simulink model "sm_tVtest_belt_trackSeg"  (R2026a)
settings: Solver=ode23t  StopTime=2.5  AbsTol=1e-3  EnableMultiTasking=on
undefined symbols (not defined in the file or in its folder): Trac, track_seg_tgts_seg25i2u0r3, X, Y, Z
libraries: sm_lib x9, sm_trackV_lib_belt_contact_internal_sets x3, sm_trackV_lib_belt_contact x3, sm_trackV_lib_belt_underc_elem x3, sm_trackV_lib_belt_segment x3, nesl_utility x1
Description:
  | Belt Track Segments
  | Copyright 2024-2026 The MathWorks, Inc.
settings Model: Creator=smiller  LastModifiedBy=smiller
settings DebuggingCC: SubsystemReferenceDiagnosticForUnitTest=warning
settings SimscapeCC: SimscapeNominalValues="[{\"value\":\"1\",\"unit\":\"A\"},{\"value\":\"1\",\"unit\":\"bar\"},{\"value\":\"1\",\"unit\":\"cm^2\"},{\"value\":\"1\",\"unit\":\"cm^3/s\"},{\"value\":\"1\",\"unit\":\"kJ/kg\"},{\"value\":\"1\",\"unit\":\"kW\"},{\"value\":\"1\",\"unit\":\"l\"},{\"value\":\"1\",\"unit\":\"N\"},{\"value\":\"1\",\"unit\":\"N*m\"},{\"value\":\"1\",\"unit\":\"V\"}]"  SimscapeLogSimulationStatistics=on
settings ExplorerConfigSet: InternalSimMechanicsExplorerSettings="<ExplorerConfiguration><canonicalview>default</canonicalview><AnimationSetting><BasePlaybackSpeed>1.0</BasePlaybackSpeed><PlaybackSpeedFactor>1.0</PlaybackSpeedFactor></AnimationSetting><TilePanel><TileInfo><Tiles Columns=\"1\" Count=\"1\" Rows=\"1\"><Column Weight=\"1\"/><Row Weight=\"1\"/><Tile Height=\"1\" Width=\"1\" X=\"0\" Y=\"0\"/></Tiles></TileInfo><SceneInfo><SceneViewer><BGColor><R>1</R><G>1</G><B>1</B></BGColor><Camera><DoPerspective>off</DoPerspective><Position><X>0.0792342818112368175</X><Y>-1.47217004076199931</Y><Z>-0.215028231058741581</Z></Position><Center><X>-0.384436321912249857</X><Y>-0.0022500717732171216</Y><Z>-0.342061483853710324</Z></Center><Up><X>0.00408619380834399082</X><Y>0.0873795501498821903</Y><Z>0.996166711567780361</Z></Up><ViewLimDist>1</ViewLimDist><YLim>0.935866935253143351</YLim><XLim>1.10917562696668837</XLim></Camera></SceneViewer></SceneInfo></TilePanel><MechEditorPanel><Cameras/><GfxPanelCameraMap/><VideoCreator><PlaybackSpeedRatio>1.0</PlaybackSpeedRatio><FrameRate>30</FrameRate><VideoFormat>Motion JPEG AVI</VideoFormat><FrameSize>auto</FrameSize></VideoCreator></MechEditorPanel></ExplorerConfiguration>"

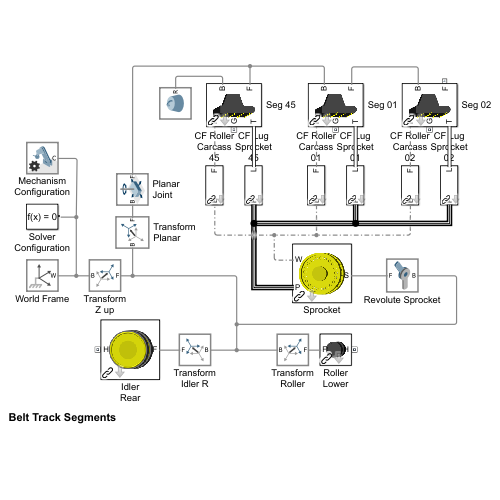
[thumbnail: Simulink's stored preview of the top-level diagram]
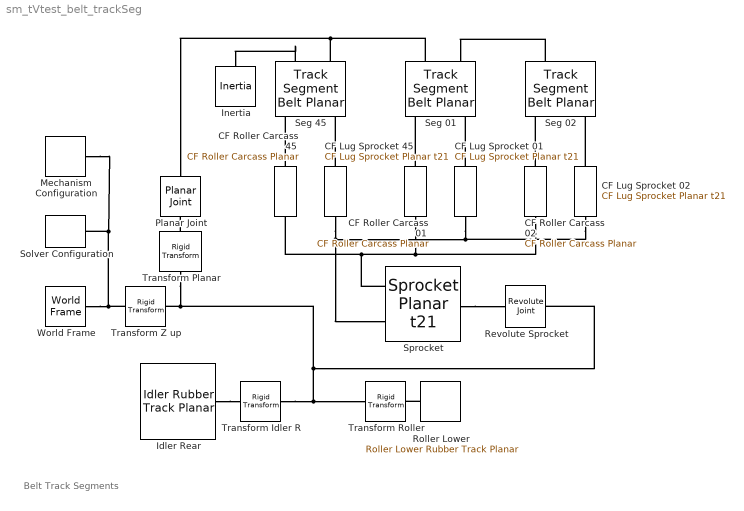
== system sm_tVtest_belt_trackSeg ==
  note: Belt Track Segments
  CF Lug Sprocket 01 : sm_trackV_lib_belt_contact_internal_sets/CF Lug Sprocket Planar t21  K_SprocketLug=Trac.Contact.SprocketLug.K  B_SprocketLug=Trac.Contact.SprocketLug.B  TW_SprocketLug=Trac.Contact.SprocketLug.TW
  CF Lug Sprocket 02 : sm_trackV_lib_belt_contact_internal_sets/CF Lug Sprocket Planar t21  K_SprocketLug=Trac.Contact.SprocketLug.K  B_SprocketLug=Trac.Contact.SprocketLug.B  TW_SprocketLug=Trac.Contact.SprocketLug.TW
  CF Lug Sprocket 45 : sm_trackV_lib_belt_contact_internal_sets/CF Lug Sprocket Planar t21  K_SprocketLug=Trac.Contact.SprocketLug.K  B_SprocketLug=Trac.Contact.SprocketLug.B  TW_SprocketLug=Trac.Contact.SprocketLug.TW
  CF Roller Carcass 01 : sm_trackV_lib_belt_contact/CF Roller Carcass Planar  K_Roller=Trac.Contact.SprocketRoller.K  B_Roller=Trac.Contact.SprocketRoller.B  TW_Roller=Trac.Contact.SprocketRoller.TW
  CF Roller Carcass 02 : sm_trackV_lib_belt_contact/CF Roller Carcass Planar  K_Roller=Trac.Contact.SprocketRoller.K  B_Roller=Trac.Contact.SprocketRoller.B  TW_Roller=Trac.Contact.SprocketRoller.TW
  CF Roller Carcass 45 : sm_trackV_lib_belt_contact/CF Roller Carcass Planar  K_Roller=Trac.Contact.SprocketRoller.K  B_Roller=Trac.Contact.SprocketRoller.B  TW_Roller=Trac.Contact.SprocketRoller.TW
  Idler Rear : sm_trackV_lib_belt_underc_elem/Idler Rubber Track Planar  idler_rad=Trac.IdlerR.rad  idler_len=Trac.IdlerR.len  wheel_clr=Trac.IdlerR.Wheel.clr  rim_rad=Trac.IdlerR.Rim.rad  rim_hub_rad=Trac.IdlerF.Rim.hub_rad  rim_xc=Trac.IdlerR.Rim.rim_xc  idler_rho=Trac.IdlerR.rho  idler_opc=Trac.IdlerR.opc  idler_clr=Trac.IdlerR.clr  idler_axle_rad=Trac.IdlerR.Axle.rad  idler_axle_len=Trac.IdlerR.Axle.len  idler_axle_rho=Trac.IdlerR.Axle.rho  idler_axle_opc=Trac.IdlerR.Axle.opc  idler_axle_clr=Trac.IdlerR.Axle.clr  idler_contgeo_clr=Trac.IdlerR.belt_contact.clr  idler_contgeo_opc=Trac.IdlerR.belt_contact.opc
  Inertia : sm_lib/Body Elements/Inertia  InertiaType=Custom  Mass=Trac.Belt.mass  MassUnits=kg  CenterOfMass=[0 0 0]  CenterOfMassUnits=m  MomentsOfInertia=[1 1 1]  MomentsOfInertiaUnits=kg*m^2  ProductsOfInertia=[0 0 0]  ProductsOfInertiaUnits=kg*m^2  GraphicType=None  MarkerShape=Inertia  MarkerSize=20  GraphicVisPropType=SimpleVisualProperties  GraphicDiffuseColor=[0.5 0.5 0.5]  GraphicOpacity=1.0  GraphicSpecularColor=[0.5 0.5 0.5 1.0]  GraphicAmbientColor=[0.15 0.15 0.15 1.0]  GraphicEmissiveColor=[0.0 0.0 0.0 1.0]  GraphicShininess=75
  Mechanism Configuration : sm_lib/Utilities/Mechanism Configuration  UniformGravity=Constant  GravityVector=[0 0 -9.80665]  GravityVectorUnits=m/s^2  LinearizationDelta=0.001  JointModeTransitionNonlinearIterations=2
  Planar Joint : sm_lib/Joints/Planar Joint  JointMode=Normal  CompositeWrenchDir=FollowerOnBase  CompositeWrenchFrame=BaseFrame  SenseConstraintForce=off  SenseConstraintTorque=off  SenseTotalForce=off  SenseTotalTorque=off  PxPositionTargetSpecify=off  PxPositionTargetPriority=High  PxPositionTargetValue=0  PxPositionTargetValueUnits=m  PxVelocityTargetSpecify=off  PxVelocityTargetPriority=High  PxVelocityTargetValue=0  PxVelocityTargetValueUnits=m/s  PxEquilibriumPosition=0  PxEquilibriumPositionUnits=m  PxSpringStiffness=0  PxSpringStiffnessUnits=N/m  PxDampingCoefficient=0  PxDampingCoefficientUnits=N/(m/s)  PxLowerLimitSpecify=off  PxLowerLimitBound=-1  PxLowerLimitBoundUnits=m  PxLowerLimitStiffness=1e6  PxLowerLimitStiffnessUnits=N/m  PxLowerLimitDamping=1e3  PxLowerLimitDampingUnits=N/(m/s)  PxLowerLimitTransitionRegionWidth=1e-4  PxLowerLimitTransitionRegionWidthUnits=m  PxUpperLimitSpecify=off  PxUpperLimitBound=1  PxUpperLimitBoundUnits=m  PxUpperLimitStiffness=1e6  PxUpperLimitStiffnessUnits=N/m  PxUpperLimitDamping=1e3  PxUpperLimitDampingUnits=N/(m/s)  PxUpperLimitTransitionRegionWidth=1e-4  PxUpperLimitTransitionRegionWidthUnits=m  PxTorqueActuationMode=NoTorque  PxMotionActuationMode=ComputedMotion  PxSensePosition=off  PxSenseVelocity=off  PxSenseAcceleration=off  PxSenseTorqueForce=off  PxSenseLowerLimitTorqueForce=off  PxSenseUpperLimitTorqueForce=off  PyPositionTargetSpecify=off  PyPositionTargetPriority=High  PyPositionTargetValue=0  PyPositionTargetValueUnits=m  PyVelocityTargetSpecify=off  PyVelocityTargetPriority=High  PyVelocityTargetValue=0  PyVelocityTargetValueUnits=m/s  PyEquilibriumPosition=0  PyEquilibriumPositionUnits=m  PySpringStiffness=0  PySpringStiffnessUnits=N/m  PyDampingCoefficient=0  PyDampingCoefficientUnits=N/(m/s)  PyLowerLimitSpecify=off  PyLowerLimitBound=-1  PyLowerLimitBoundUnits=m  PyLowerLimitStiffness=1e6  PyLowerLimitStiffnessUnits=N/m  PyLowerLimitDamping=1e3  PyLowerLimitDampingUnits=N/(m/s)  PyLowerLimitTransitionRegionWidth=1e-4  PyLowerLimitTransitionRegionWidthUnits=m  PyUpperLimitSpecify=off  PyUpperLimitBound=1  PyUpperLimitBoundUnits=m  PyUpperLimitStiffness=1e6  PyUpperLimitStiffnessUnits=N/m  PyUpperLimitDamping=1e3  PyUpperLimitDampingUnits=N/(m/s)  PyUpperLimitTransitionRegionWidth=1e-4  PyUpperLimitTransitionRegionWidthUnits=m  PyTorqueActuationMode=NoTorque  PyMotionActuationMode=ComputedMotion  PySensePosition=off  PySenseVelocity=off  PySenseAcceleration=off  PySenseTorqueForce=off  PySenseLowerLimitTorqueForce=off  PySenseUpperLimitTorqueForce=off  RzPositionTargetSpecify=on  RzPositionTargetPriority=High  RzPositionTargetValue=0  RzPositionTargetValueUnits=deg  RzVelocityTargetSpecify=off  RzVelocityTargetPriority=High  RzVelocityTargetValue=0  RzVelocityTargetValueUnits=deg/s  RzEquilibriumPosition=0  RzEquilibriumPositionUnits=deg  RzSpringStiffness=0  RzSpringStiffnessUnits=N*m/deg  RzDampingCoefficient=0  RzDampingCoefficientUnits=N*m/(deg/s)  RzLowerLimitSpecify=off  RzLowerLimitBound=-90  RzLowerLimitBoundUnits=deg  RzLowerLimitStiffness=1e4  RzLowerLimitStiffnessUnits=N*m/deg  RzLowerLimitDamping=10  RzLowerLimitDampingUnits=N*m/(deg/s)  RzLowerLimitTransitionRegionWidth=0.1  RzLowerLimitTransitionRegionWidthUnits=deg  RzUpperLimitSpecify=off  RzUpperLimitBound=90  RzUpperLimitBoundUnits=deg  RzUpperLimitStiffness=1e4  RzUpperLimitStiffnessUnits=N*m/deg  RzUpperLimitDamping=10  RzUpperLimitDampingUnits=N*m/(deg/s)  RzUpperLimitTransitionRegionWidth=0.1  RzUpperLimitTransitionRegionWidthUnits=deg  RzTorqueActuationMode=NoTorque  RzMotionActuationMode=ComputedMotion  RzSensePosition=off  RzSenseVelocity=off  RzSenseAcceleration=off  RzSenseTorqueForce=off  RzSenseLowerLimitTorqueForce=off  RzSenseUpperLimitTorqueForce=off
  Revolute Sprocket : sm_lib/Joints/Revolute Joint  JointMode=Normal  CompositeWrenchDir=FollowerOnBase  CompositeWrenchFrame=BaseFrame  SenseConstraintForce=off  SenseConstraintTorque=off  SenseTotalForce=off  SenseTotalTorque=off  PositionTargetSpecify=off  PositionTargetPriority=High  PositionTargetValue=0  PositionTargetValueUnits=deg  VelocityTargetSpecify=off  VelocityTargetPriority=High  VelocityTargetValue=0  VelocityTargetValueUnits=deg/s  EquilibriumPosition=0  EquilibriumPositionUnits=deg  SpringStiffness=0  SpringStiffnessUnits=N*m/deg  DampingCoefficient=0  DampingCoefficientUnits=N*m/(deg/s)  LowerLimitSpecify=off  LowerLimitBound=-90  LowerLimitBoundUnits=deg  LowerLimitStiffness=1e4  LowerLimitStiffnessUnits=N*m/deg  LowerLimitDamping=10  LowerLimitDampingUnits=N*m/(deg/s)  LowerLimitTransitionRegionWidth=0.1  LowerLimitTransitionRegionWidthUnits=deg  UpperLimitSpecify=off  UpperLimitBound=90  UpperLimitBoundUnits=deg  UpperLimitStiffness=1e4  UpperLimitStiffnessUnits=N*m/deg  UpperLimitDamping=10  UpperLimitDampingUnits=N*m/(deg/s)  UpperLimitTransitionRegionWidth=0.1  UpperLimitTransitionRegionWidthUnits=deg  TorqueActuationMode=NoTorque  MotionActuationMode=ComputedMotion  SensePosition=off  SenseVelocity=off  SenseAcceleration=off  SenseTorqueForce=off  SenseLowerLimitTorqueForce=off  SenseUpperLimitTorqueForce=off
  Roller Lower : sm_trackV_lib_belt_underc_elem/Roller Lower Rubber Track Planar  roller_lower_rad=Trac.Roller.Lower.rad  roller_lower_len=Trac.Roller.Lower.len  roller_lower_rho=Trac.Roller.Lower.rho  roller_lower_clr=Trac.Roller.Lower.clr  roller_lower_opc=Trac.Roller.Lower.opc  roller_lower_rim_thk=Trac.Roller.Lower.rim_thk  roller_lower_rim_len=Trac.Roller.Lower.rim_len  roller_lower_axle_rad=Trac.Roller.Lower.Axle.rad  roller_lower_axle_len=Trac.Roller.Lower.Axle.len  roller_lower_axle_rho=Trac.Roller.Lower.Axle.rho  roller_lower_axle_opc=Trac.Roller.Lower.Axle.opc  roller_lower_axle_clr=Trac.Roller.Lower.Axle.clr  roller_lower_contgeo_clr=Trac.Roller.Lower.belt_contact.clr  roller_lower_contgeo_opc=Trac.Roller.Lower.belt_contact.opc
  Seg 01 : sm_trackV_lib_belt_segment/Track Segment Belt Planar  carc_len=Trac.Belt.l  carc_wid=Trac.Belt.w  carc_thk=Trac.Belt.pad_h  carc_mass=Trac.Belt.mass  carc_cg=Trac.Belt.cg  carc_moi=Trac.Belt.moi  carc_poi=Trac.Belt.poi  carc_clr=Trac.Belt.clr  carc_opc=Trac.Belt.opc  lug_hei=Trac.Belt.Lug.h  lug_lb=Trac.Belt.Lug.lb  lug_lt=Trac.Belt.Lug.lt  lug_w=Trac.Belt.Lug.w  lug_xc=Trac.Belt.Lug.xc  lug_clr=Trac.Belt.clr  lug_opc=Trac.Belt.opc*0.5  posTgtSpecify=on  posTgtPriority=High  PositionTargetValue=track_seg_tgts_seg25i2u0r3{1,3}  DampingCoefficient=Trac.Belt.damping  lug_line_clr=Trac.Belt.lug_contact.clr  lug_line_opc=Trac.Belt.lug_contact.opc  carc_line_clr=Trac.Belt.carcass_contact.clr  carc_line_opc=Trac.Belt.carcass_contact.opc  ptcld_belt=Trac.Belt.ground_contact.ptcld.pts  ptcld_belt_rad=Trac.Belt.ground_contact.ptcld.rad  ptcld_belt_clr=Trac.Belt.ground_contact.ptcld.clr  ptcld_belt_opc=Trac.Belt.ground_contact.ptcld.opc
  Seg 02 : sm_trackV_lib_belt_segment/Track Segment Belt Planar  carc_len=Trac.Belt.l  carc_wid=Trac.Belt.w  carc_thk=Trac.Belt.pad_h  carc_mass=Trac.Belt.mass  carc_cg=Trac.Belt.cg  carc_moi=Trac.Belt.moi  carc_poi=Trac.Belt.poi  carc_clr=Trac.Belt.clr  carc_opc=Trac.Belt.opc  lug_hei=Trac.Belt.Lug.h  lug_lb=Trac.Belt.Lug.lb  lug_lt=Trac.Belt.Lug.lt  lug_w=Trac.Belt.Lug.w  lug_xc=Trac.Belt.Lug.xc  lug_clr=Trac.Belt.clr  lug_opc=Trac.Belt.opc*0.5  posTgtSpecify=on  posTgtPriority=High  PositionTargetValue=track_seg_tgts_seg25i2u0r3{2,3}  DampingCoefficient=Trac.Belt.damping  lug_line_clr=Trac.Belt.lug_contact.clr  lug_line_opc=Trac.Belt.lug_contact.opc  carc_line_clr=Trac.Belt.carcass_contact.clr  carc_line_opc=Trac.Belt.carcass_contact.opc  ptcld_belt=Trac.Belt.ground_contact.ptcld.pts  ptcld_belt_rad=Trac.Belt.ground_contact.ptcld.rad  ptcld_belt_clr=Trac.Belt.ground_contact.ptcld.clr  ptcld_belt_opc=Trac.Belt.ground_contact.ptcld.opc
  Seg 45 : sm_trackV_lib_belt_segment/Track Segment Belt Planar  carc_len=Trac.Belt.l  carc_wid=Trac.Belt.w  carc_thk=Trac.Belt.pad_h  carc_mass=Trac.Belt.mass  carc_cg=Trac.Belt.cg  carc_moi=Trac.Belt.moi  carc_poi=Trac.Belt.poi  carc_clr=Trac.Belt.clr  carc_opc=Trac.Belt.opc  lug_hei=Trac.Belt.Lug.h  lug_lb=Trac.Belt.Lug.lb  lug_lt=Trac.Belt.Lug.lt  lug_w=Trac.Belt.Lug.w  lug_xc=Trac.Belt.Lug.xc  lug_clr=Trac.Belt.clr  lug_opc=Trac.Belt.opc*0.5  posTgtSpecify=on  posTgtPriority=High  PositionTargetValue=track_seg_tgts_seg25i2u0r3{45,3}  DampingCoefficient=Trac.Belt.damping  lug_line_clr=Trac.Belt.lug_contact.clr  lug_line_opc=Trac.Belt.lug_contact.opc  carc_line_clr=Trac.Belt.carcass_contact.clr  carc_line_opc=Trac.Belt.carcass_contact.opc  ptcld_belt=Trac.Belt.ground_contact.ptcld.pts  ptcld_belt_rad=Trac.Belt.ground_contact.ptcld.rad  ptcld_belt_clr=Trac.Belt.ground_contact.ptcld.clr  ptcld_belt_opc=Trac.Belt.ground_contact.ptcld.opc
  Solver Configuration : nesl_utility/Solver Configuration  PhysicalDomain=network_engine_domain  SubClassName=solver  LeftPortType=input  RightPortType=generic  Tones=[]  Harmonics=[]  SimulateNoise=off  Profile=off  UseLocalSampling=off  EnableSwitchedLinearOptims=on  FrequencyDomain=off  UseCCode=off  RelTol=0.001  AbsTol=1e-06  MinStep=1e-09  ToWorkspace=off  RevertToSquareIcSolve=off  NumHomotopyIterations=100  PhasorMode=off  PhasorModeNumHarmonics=1  ConsistencySolver=NEWTON_XTOL_AFTER_FTOL  CanonicalOrdering=UNORDERED  OptimizeIntermediates=UNOPTIMIZED  IndexReductionMethod=DerivativeReplacement  DoDC=off  ResidualTolerance=1e-09  ConsistencyTolSource=GLOBAL  ConsistencyAbsTol=0.001  ConsistencyRelTol=0.001  ConsistencyTolFactor=0.001  UseLocalSolver=off  LocalSolverChoice=NE_BACKWARD_EULER_ADVANCER  ResolveIndetEquations=on  FunctionEvalNumThread=1  LocalSolverSampleTime=0.001  DoFixedCost=off  MaxNonlinIter=3  MaxModeIter=2  ComputeImpulses=off  ImpulseIterations=2  LinearAlgebra=Sparse  LinearAlgebraNumThread=0  EquationFormulation=NE_TIME_EF  DelaysMemoryBudget=1024  AutomaticFiltering=on  FilteringTimeConstant=0.001  PartitionStorageMethod=AS_NEEDED  PartitionMemoryBudget=1024  PartitionMethod=FAST  MultibodyUseLocalSolver=off  MultibodyLocalSolverChoice=ODE1  MultibodyLocalSolverSampleTime=0.001
  Sprocket : sm_trackV_lib_belt_underc_elem/Sprocket Planar t21  sprk_wid_roll=Trac.Sprocket.Roller.wid  sprk_rad_roll=Trac.Sprocket.Roller.rad  sprk_opc=Trac.Sprocket.Roller.opc  sprk_clr=Trac.Sprocket.Roller.clr  sprk_rad_pitch=Trac.Sprocket.Spoke.pitch_rad  sprk_spoke_rad=Trac.Sprocket.Spoke.rad  sprk_spoke_len=Trac.Sprocket.Spoke.len  sprk_spoke_num=Trac.Sprocket.nSpokes  sprk_spoke_clr=Trac.Sprocket.Spoke.clr  sprk_spoke_opc=Trac.Sprocket.Spoke.opc  rim_spoke_xc=Trac.Sprocket.Rim.spoke_xc  rim_thk=Trac.Sprocket.Rim.thk  rim_ir=Trac.Sprocket.Rim.rad_inner  sprk_contgeo_roller_clr=Trac.Sprocket.roller_contact.clr  sprk_contgeo_roller_opc=Trac.Sprocket.roller_contact.opc  sprk_contgeo_spoke_clr=Trac.Sprocket.spoke_contact.clr  sprk_contgeo_spoke_opc=Trac.Sprocket.spoke_contact.opc
  Transform Idler R : sm_lib/Frames and Transforms/Rigid Transform  RotationMethod=None  FollAlignAxisA=+X  BaseAlignAxisA=+Y  FollAlignAxisB=+Y  BaseAlignAxisB=+Z  RotationStandardAxis=+Z  RotationAngle=0.0  RotationAngleUnits=deg  RotationArbitraryAxis=[0 0 1]  RotationSequenceAxes=FollowerAxes  RotationSequence=XYX  RotationSequenceAngles=[0 0 0]  RotationSequenceAnglesUnits=deg  RotationMatrix=[1 0 0; 0 1 0; 0 0 1]  Quaternion=[1 0 0 0]  TranslationMethod=Cartesian  TranslationCartesianOffset=[Trac.Frame.SprkOffLon.IdlerR -Trac.Frame.SprkOffVer.IdlerR 0]  TranslationCartesianOffsetUnits=m  TranslationStandardAxis=+X  TranslationStandardOffset=1  TranslationStandardOffsetUnits=m  TranslationROffset=0  TranslationROffsetUnits=m  TranslationThetaOffset=0  TranslationThetaOffsetUnits=deg  TranslationZOffset=0  TranslationZOffsetUnits=m
  Transform Planar : sm_lib/Frames and Transforms/Rigid Transform  RotationMethod=StandardAxis  FollAlignAxisA=+X  BaseAlignAxisA=+Y  FollAlignAxisB=+Y  BaseAlignAxisB=+Z  RotationStandardAxis=+Z  RotationAngle=-track_seg_tgts_seg25i2u0r3{1,3}/2  RotationAngleUnits=deg  RotationArbitraryAxis=[0 0 1]  RotationSequenceAxes=FollowerAxes  RotationSequence=XYX  RotationSequenceAngles=[0 0 0]  RotationSequenceAnglesUnits=deg  RotationMatrix=[1 0 0; 0 1 0; 0 0 1]  Quaternion=[1 0 0 0]  TranslationMethod=StandardAxis  TranslationCartesianOffset=[0 0 0]  TranslationCartesianOffsetUnits=m  TranslationStandardAxis=+Y  TranslationStandardOffset=-Trac.Sprocket.Roller.rad-Trac.Belt.pad_h/2  TranslationStandardOffsetUnits=m  TranslationROffset=0  TranslationROffsetUnits=m  TranslationThetaOffset=0  TranslationThetaOffsetUnits=deg  TranslationZOffset=0  TranslationZOffsetUnits=m
  Transform Roller : sm_lib/Frames and Transforms/Rigid Transform  RotationMethod=None  FollAlignAxisA=+X  BaseAlignAxisA=+Y  FollAlignAxisB=+Y  BaseAlignAxisB=+Z  RotationStandardAxis=+Z  RotationAngle=0.0  RotationAngleUnits=deg  RotationArbitraryAxis=[0 0 1]  RotationSequenceAxes=FollowerAxes  RotationSequence=XYX  RotationSequenceAngles=[0 0 0]  RotationSequenceAnglesUnits=deg  RotationMatrix=[1 0 0; 0 1 0; 0 0 1]  Quaternion=[1 0 0 0]  TranslationMethod=Cartesian  TranslationCartesianOffset=[Trac.Frame.SprkOffLon.Lower(2) -Trac.Frame.SprkOffVer.Lower 0]  TranslationCartesianOffsetUnits=m  TranslationStandardAxis=+X  TranslationStandardOffset=-1  TranslationStandardOffsetUnits=m  TranslationROffset=0  TranslationROffsetUnits=m  TranslationThetaOffset=0  TranslationThetaOffsetUnits=deg  TranslationZOffset=0  TranslationZOffsetUnits=m
  Transform Z up : sm_lib/Frames and Transforms/Rigid Transform  RotationMethod=StandardAxis  FollAlignAxisA=+X  BaseAlignAxisA=+Y  FollAlignAxisB=+Y  BaseAlignAxisB=+Z  RotationStandardAxis=+X  RotationAngle=-90  RotationAngleUnits=deg  RotationArbitraryAxis=[0 0 1]  RotationSequenceAxes=FollowerAxes  RotationSequence=XYX  RotationSequenceAngles=[0 0 0]  RotationSequenceAnglesUnits=deg  RotationMatrix=[1 0 0; 0 1 0; 0 0 1]  Quaternion=[1 0 0 0]  TranslationMethod=None  TranslationCartesianOffset=[0 0 0]  TranslationCartesianOffsetUnits=m  TranslationStandardAxis=+Z  TranslationStandardOffset=0  TranslationStandardOffsetUnits=m  TranslationROffset=0  TranslationROffsetUnits=m  TranslationThetaOffset=0  TranslationThetaOffsetUnits=deg  TranslationZOffset=0  TranslationZOffsetUnits=m
  World Frame : sm_lib/Frames and Transforms/World Frame
  connections:
  Seg 02/LConn1 -- Seg 01/LConn2
  Idler Rear/LConn1 -- Transform Idler R/RConn1
  Transform Idler R/LConn1 -- Transform Roller/LConn1 -- Transform Planar/LConn1 -- Transform Z up/RConn1 -- Revolute Sprocket/LConn1
  Roller Lower/LConn1 -- Transform Roller/RConn1
  Seg 01/LConn1 -- Seg 45/LConn2 -- Planar Joint/RConn1
  Transform Planar/RConn1 -- Planar Joint/LConn1
  CF Lug Sprocket 02/LConn1 -- Sprocket/LConn1 -- CF Lug Sprocket 45/LConn1 -- CF Lug Sprocket 01/LConn1
  CF Lug Sprocket 02/RConn1 -- Seg 02/RConn3
  CF Lug Sprocket 01/RConn1 -- Seg 01/RConn3
  CF Lug Sprocket 45/RConn1 -- Seg 45/RConn3
  CF Roller Carcass 02/LConn1 -- Sprocket/LConn2 -- CF Roller Carcass 45/LConn1 -- CF Roller Carcass 01/LConn1
  CF Roller Carcass 01/RConn1 -- Seg 01/RConn1
  CF Roller Carcass 02/RConn1 -- Seg 02/RConn1
  CF Roller Carcass 45/RConn1 -- Seg 45/RConn1
  Seg 45/LConn1 -- Inertia/RConn1
  Transform Z up/LConn1 -- Mechanism Configuration/RConn1 -- Solver Configuration/RConn1 -- World Frame/RConn1
  Sprocket/RConn1 -- Revolute Sprocket/RConn1
